simulink model "simdycmodel"  (R2018a)
settings: Solver=FixedStepAuto  StartTime=0.0  StopTime=10.0  RelTol=1e-3
values from neighbouring files (symbols this model uses):
  a11 = -2*(cf+cr)/m/v    (= -9.36)    [dyc.m]    (also in dyc_obs.m; normal_vehicle.m)
  a12 = -1-2*(lf*cf-lr*cr)/m/v/v    (= -0.9745984)    [dyc.m]    (also in dyc_obs.m; normal_vehicle.m)
  a21 = -2*(lf*cf-lr*cr)/iz    (= 12.3270440252)    [dyc.m]    (also in dyc_obs.m; normal_vehicle.m)
  a22 = -2*(lf*lf*cf+lr*lr*cr)/iz/v    (= -9.16473962264)    [dyc.m]    (also in dyc_obs.m; normal_vehicle.m)
  b11 = 2*cf/m/v    (= 3.6)    [dyc.m]    (also in dyc_obs.m; normal_vehicle.m)
  b12 = 0    [dyc.m]    (also in dyc_obs.m)
  b21 = 2*lf*cf/iz    (= 94.3396226415)    [dyc.m]    (also in dyc_obs.m; normal_vehicle.m)
  b22 = 1/iz    (= 0.0062893081761)    [dyc.m]    (also in dyc_obs.m)
  G = input('Without Control (0) or With DYC Control (1) : ')    [dyc.m]    (also in dyc_obs.m)
  Kb = Kfb(1,1)    [dyc.m]    (also in dyc_obs.m)
  kbeta = 0    [dyc.m]    (also in dyc_obs.m)
  Kff = (a22*b11-a12*b21)/(a12*b22*n)    (= -514.298169648)    [dyc.m]    (also in dyc_obs.m)
  Kg = Kfb(1,2)    [dyc.m]    (also in dyc_obs.m)
  kgamma = -b11/a12/n    (= 0.197530971715)    [dyc.m]    (also in dyc_obs.m)
  mydt = 0.01    [dyc.m]    (also in dyc_obs.m; normal_vehicle.m)
  n = 18.7    [dyc.m]    (also in dyc_obs.m; normal_vehicle.m)
  tbeta = 0.05    [dyc.m]    (also in dyc_obs.m)
  tgamma = 0.05    [dyc.m]    (also in dyc_obs.m)
settings Model: Creator=aoki-soya  LastModifiedBy=aoki-soya

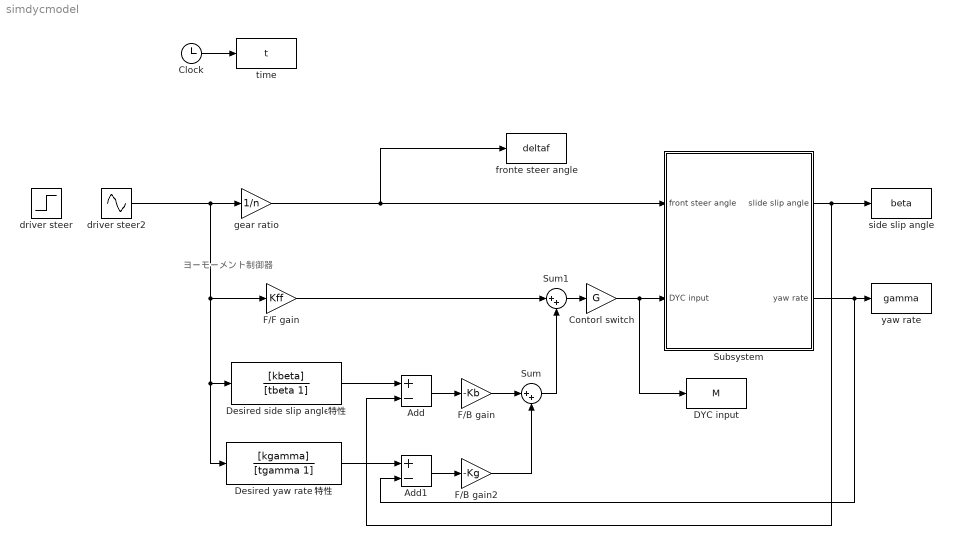
== system simdycmodel ==
  note: ヨーモーメント制御器
  Add : Sum  Inputs=+-
  Add1 : Sum  Inputs=+-
  Clock : Clock
      settings: Decimation=1/mydt
  Contorl switch : Gain  Gain=G
  DYC input : ToWorkspace  VariableName=M  SaveFormat=Timeseries  SampleTime=-1
  Desired side slip angle特性 : TransferFcn  Numerator=[kbeta]  Denominator=[tbeta 1]
  Desired yaw rate 特性 : TransferFcn  Numerator=[kgamma]  Denominator=[tgamma 1]
  F/B gain : Gain  Gain=-Kb
  F/B gain2 : Gain  Gain=-Kg
  F/F gain : Gain  Gain=Kff
  Subsystem : Subsystem
  Sum : Sum  Inputs=|++
  Sum1 : Sum  Inputs=|++
  driver steer : Step  After=15*pi/180  SampleTime=mydt
  driver steer2 : Sin  SampleTime=mydt
  fronte steer angle : ToWorkspace  VariableName=deltaf  SaveFormat=Timeseries  SampleTime=-1
  gear ratio : Gain  Gain=1/n
  side slip angle : ToWorkspace  VariableName=beta  SaveFormat=Timeseries  SampleTime=-1
  time : ToWorkspace  VariableName=t  SaveFormat=Timeseries  SampleTime=-1
  yaw rate : ToWorkspace  VariableName=gamma  SaveFormat=Timeseries  SampleTime=-1
  wires:
  Clock/1 -> time/1
  driver steer2/1 -> Desired yaw rate 特性/1, Desired side slip angle特性/1, F/F gain/1, gear ratio/1
  gear ratio/1 -> fronte steer angle/1, Subsystem/1(front steer angle)
  Subsystem/1(slide slip angle) -> side slip angle/1, Add/2
  Subsystem/2(yaw rate) -> Add1/2, yaw rate/1
  Desired side slip angle特性/1 -> Add/1
  Desired yaw rate 特性/1 -> Add1/1
  Add/1 -> F/B gain/1
  Add1/1 -> F/B gain2/1
  F/B gain/1 -> Sum/1
  F/B gain2/1 -> Sum/2
  F/F gain/1 -> Sum1/1
  Sum/1 -> Sum1/2
  Sum1/1 -> Contorl switch/1
  Contorl switch/1 -> Subsystem/2(DYC input), DYC input/1

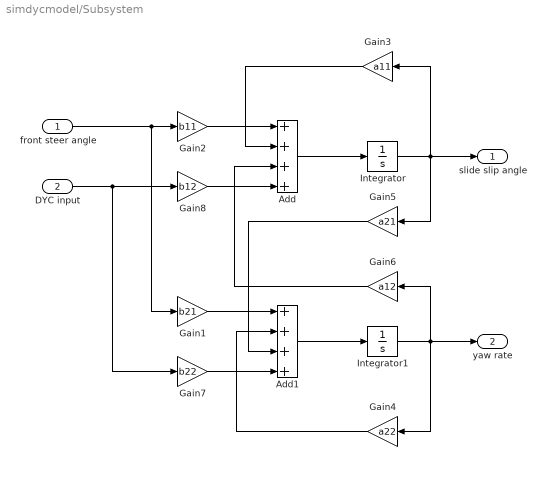
== system simdycmodel/Subsystem ==
  front steer angle : Inport
  DYC input : Inport  Port=2
  Add : Sum  Inputs=++++
  Add1 : Sum  Inputs=++++
  Gain1 : Gain  Gain=b21
  Gain2 : Gain  Gain=b11
  Gain3 : Gain  Gain=a11
  Gain4 : Gain  Gain=a22
  Gain5 : Gain  Gain=a21
  Gain6 : Gain  Gain=a12
  Gain7 : Gain  Gain=b22
  Gain8 : Gain  Gain=b12
  Integrator : Integrator
  Integrator1 : Integrator
  slide slip angle : Outport
  yaw rate : Outport  Port=2
  wires:
  Add1/1 -> Integrator1/1
  Integrator1/1 -> yaw rate/1, Gain6/1, Gain4/1
  Gain1/1 -> Add1/1
  Gain5/1 -> Add1/3
  Integrator/1 -> slide slip angle/1, Gain5/1, Gain3/1
  front steer angle/1 -> Gain1/1, Gain2/1
  Gain2/1 -> Add/1
  Gain4/1 -> Add1/2
  Add/1 -> Integrator/1
  Gain6/1 -> Add/3
  Gain3/1 -> Add/2
  DYC input/1 -> Gain7/1, Gain8/1
  Gain8/1 -> Add/4
  Gain7/1 -> Add1/4
